simulink model "modelo_q1_fk"  (R2016a)
settings: Solver=VariableStepAuto  StartTime=0.0  StopTime=20  MaxStep=0.001  RelTol=1e-3
values from neighbouring files (symbols this model uses):
  Cm = [1 0 0; 0 1 0]    [gazebo_parameters.m]    (also in gpc.m = [C zeros(ny,1)]; kalman_filter.m)
  Dmsim = zeros(2,1)    [gazebo_parameters.m]    (also in kalman_filter.m = zeros(2,2))
  Kd = dlqr(Amd, Bmd,eye(3),0.7)    [gazebo_parameters.m]    (also in gpc.m = dlqr(A, B, eye(3),1); kalman_filter.m; questao1.m = dlqr(Ad,Bd,Q,R))
  Lkf = dlqr(Amd',Cm',1e-4*eye(3),1*eye(2))'    [gazebo_parameters.m]    (also in kalman_filter.m)
  Pam = 1e8*eye(3)    [gazebo_parameters.m]    (also in kalman_filter.m = 1e-6*eye(3))
  Tsm = 0.005    [gazebo_parameters.m]    (also in kalman_filter.m)
  v = [v1 v2]'    [controledesacoplante.m]    (also in gazebo_parameters.m = 1e-7*eye(2); kalman_filter.m = 1e-8*eye(2); v(1,1) = 1e-0*v(1,1); v(2,2) = 1e-0*v(2,2))
  w = 1e-4*eye(3)    [gazebo_parameters.m]    (also in kalman_filter.m = 1e-10*eye(3); w(1,1) = 1e-0*w(1,1); w(2,2) = 1e-0*w(2,2); w()
  x0m = [0 0 0]    [gazebo_parameters.m]    (also in kalman_filter.m)
undefined symbols (not defined in the file or in its folder): Amd, Bmd, Discrete, sigbuilder_block, Time
libraries: simulink x10, ctrlSharedLib x1
settings Model: Creator=Regner  LastModifiedBy=Regner

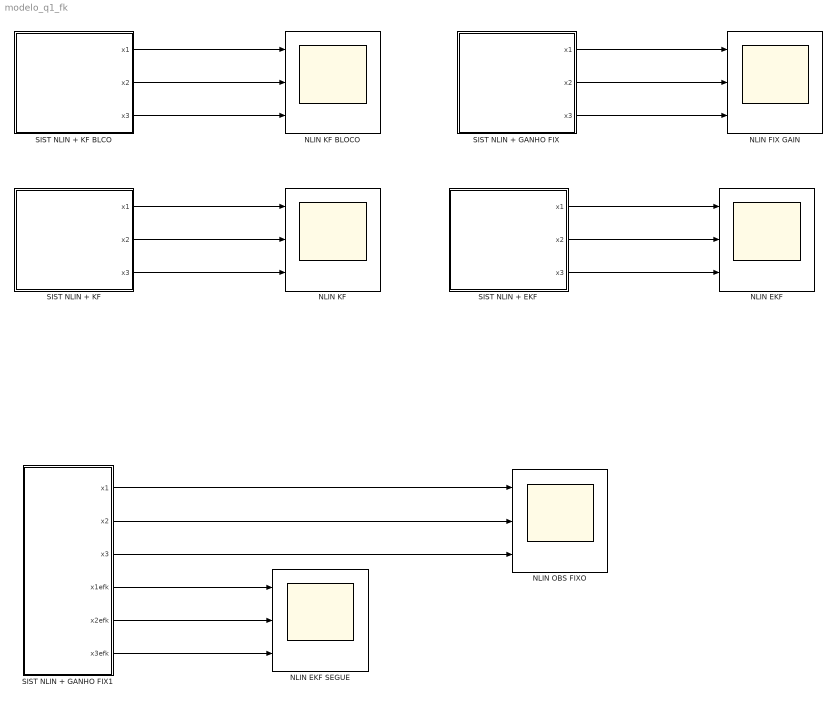
== system modelo_q1_fk ==
  NLIN EKF : Scope  NumInputPorts=3
  NLIN EKF SEGUE : Scope  NumInputPorts=3
  NLIN FIX GAIN : Scope  NumInputPorts=3
  NLIN KF : Scope  NumInputPorts=3
  NLIN KF BLOCO : Scope  NumInputPorts=3
  NLIN OBS FIXO : Scope  NumInputPorts=3
  SIST NLIN + EKF : Subsystem
  SIST NLIN + GANHO FIX : Subsystem
  SIST NLIN + GANHO FIX1 : Subsystem
  SIST NLIN + KF : Subsystem
  SIST NLIN + KF BLCO : Subsystem
  wires:
  SIST NLIN + KF/1(x1) -> NLIN KF/1
  SIST NLIN + KF/2(x2) -> NLIN KF/2
  SIST NLIN + KF/3(x3) -> NLIN KF/3
  SIST NLIN + KF BLCO/1(x1) -> NLIN KF BLOCO/1
  SIST NLIN + KF BLCO/2(x2) -> NLIN KF BLOCO/2
  SIST NLIN + KF BLCO/3(x3) -> NLIN KF BLOCO/3
  SIST NLIN + GANHO FIX/1(x1) -> NLIN FIX GAIN/1
  SIST NLIN + GANHO FIX/2(x2) -> NLIN FIX GAIN/2
  SIST NLIN + GANHO FIX/3(x3) -> NLIN FIX GAIN/3
  SIST NLIN + EKF/2(x2) -> NLIN EKF/2
  SIST NLIN + EKF/3(x3) -> NLIN EKF/3
  SIST NLIN + EKF/1(x1) -> NLIN EKF/1
  SIST NLIN + GANHO FIX1/1(x1) -> NLIN OBS FIXO/1
  SIST NLIN + GANHO FIX1/2(x2) -> NLIN OBS FIXO/2
  SIST NLIN + GANHO FIX1/3(x3) -> NLIN OBS FIXO/3
  SIST NLIN + GANHO FIX1/4(x1efk) -> NLIN EKF SEGUE/1
  SIST NLIN + GANHO FIX1/5(x2efk) -> NLIN EKF SEGUE/2
  SIST NLIN + GANHO FIX1/6(x3efk) -> NLIN EKF SEGUE/3

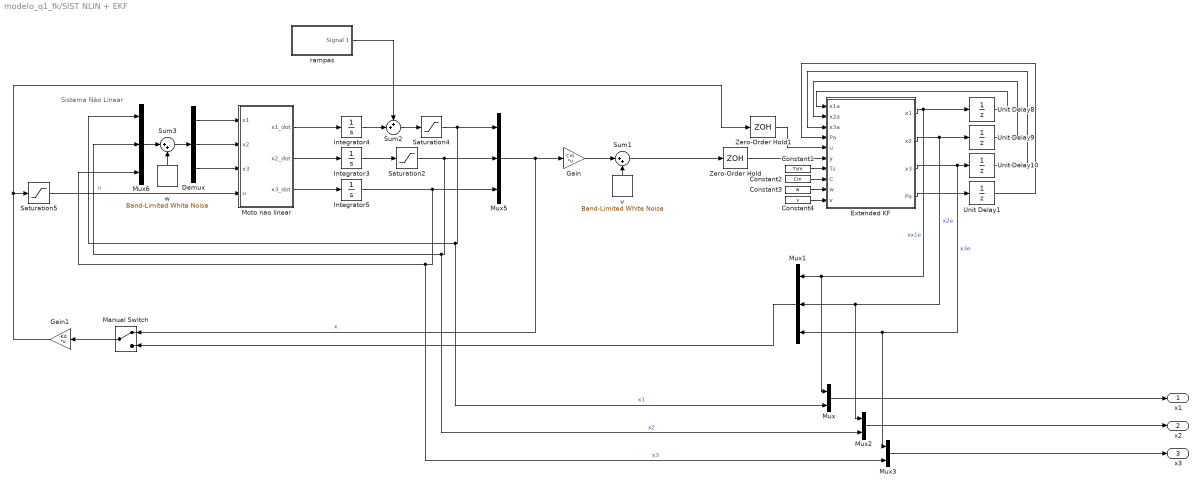
== system modelo_q1_fk/SIST NLIN + EKF ==
  note: Sistema Não Linear
  Constant1 : Constant  Value=Tsm
  Constant2 : Constant  Value=Cm
  Constant3 : Constant  Value=w
  Constant4 : Constant  Value=v
  Demux : Demux  Outputs=3
  Extended KF : MATLAB Function  TreatAsAtomicUnit=on
  Gain : Gain  Gain=Cm  Multiplication=Matrix(K*u)
  Gain1 : Gain  Gain=-Kd  Multiplication=Matrix(K*u)
  Integrator3 : Integrator  InitialCondition=x0m(2)
  Integrator4 : Integrator  InitialCondition=x0m(1)
  Integrator5 : Integrator  InitialCondition=x0m(3)
  Manual Switch : ManualSwitch
  Moto nao linear : MATLAB Function  TreatAsAtomicUnit=on
  Mux : Mux  Inputs=2
  Mux1 : Mux  Inputs=3
  Mux2 : Mux  Inputs=2
  Mux3 : Mux  Inputs=2
  Mux5 : Mux  Inputs=3
  Mux6 : Mux  Inputs=3
  Saturation2 : Saturate  UpperLimit=pi/4  LowerLimit=-pi/4
  Saturation4 : Saturate  UpperLimit=pi/4  LowerLimit=-pi/4
  Saturation5 : Saturate  UpperLimit=pi/2  LowerLimit=-pi/2
  Sum1 : Sum  Inputs=|++
  Sum2 : Sum  Inputs=++|
  Sum3 : Sum  Inputs=|++
  Unit Delay1 : UnitDelay  InitialCondition=Pam  SampleTime=Tsm
  Unit Delay10 : UnitDelay  InitialCondition=x0m(3)  SampleTime=Tsm
  Unit Delay8 : UnitDelay  InitialCondition=x0m(1)  SampleTime=Tsm
  Unit Delay9 : UnitDelay  InitialCondition=x0m(2)  SampleTime=Tsm
  Zero-Order Hold : ZeroOrderHold  SampleTime=Tsm
  Zero-Order Hold1 : ZeroOrderHold  SampleTime=Tsm
  rampas : Subsystem  Tag=STV Subsys  LoadFcn=sigbuilder_block('load');  StartFcn=sigbuilder_block('start');  StopFcn=sigbuilder_block('stop');  ClipboardFcn=sigbuilder_block('clipboard');  mask(Sigbuilder block){}
      mask help: Simulink:masks:SigbuilderBlock_MD
      mask init:
      | if ~strcmp(get_param(bdroot(gcbh),'SimulationStatus'),'stopped') tuvar = sigbuilder_block('maskInit'); end
      settings: CopyFcn=sigbuilder_block('copy');  DeleteFcn=sigbuilder_block('delete');  ModelCloseFcn=sigbuilder_block('modelClose');  PreSaveFcn=sigbuilder_block('preSave');  PauseFcn=sigbuilder_block('pause');  ContinueFcn=sigbuilder_block('continue');  NameChangeFcn=sigbuilder_block('namechange');  OpenFcn=sigbuilder_block('open',[5.4 5.4 1141.2 580.8 ]);  CloseFcn=sigbuilder_block('close');
      mask Display: plot(0, 0, 100, 100,[2, 2, 32, 32, 2], [68, 8, 8, 68, 68],[32, 2], [38, 38], [32, 19, 2],[53, 60, 44], [32, 17, 17, 2],[16, 16, 31, 31]);txt = getActiveGroup(gcbh);text(2, 100, txt,'verticalAlignment', 'top');
  v : simulink/Sources/Band-Limited White Noise  Cov=diag(v)  Ts=Tsm  seed=[23341]
  w : simulink/Sources/Band-Limited White Noise  Cov=diag(w)  Ts=Tsm  seed=[23341]
  x1 : Outport
  x2 : Outport  Port=2
  x3 : Outport  Port=3
  wires:
  Mux2/1 -> x2/1
  Gain/1 -> Sum1/1
  Constant3/1 -> Extended KF/9(w)
  v/1 -> Sum1/2
  Gain1/1 -> Saturation5/1, Zero-Order Hold1/1
  Saturation4/1 -> Mux5/1, Mux6/1, Mux/2  "x1"
  Moto nao linear/2(x2_dot) -> Integrator3/1
  Moto nao linear/1(x1_dot) -> Integrator4/1
  Moto nao linear/3(x3_dot) -> Integrator5/1
  Integrator5/1 -> Mux5/3, Mux6/3, Mux3/2  "x3"
  Sum2/1 -> Saturation4/1
  Mux5/1 -> Gain/1, Manual Switch/1  "x"
  Integrator4/1 -> Sum2/2
  Saturation5/1 -> Moto nao linear/4(u)  "u"
  Saturation2/1 -> Mux5/2, Mux6/2, Mux2/2  "x2"
  Integrator3/1 -> Saturation2/1
  rampas/1(Signal 1) -> Sum2/1
  Constant4/1 -> Extended KF/10(v)
  Mux/1 -> x1/1
  Extended KF/4(Pa) -> Unit Delay1/1
  Mux1/1 -> Manual Switch/2
  Constant2/1 -> Extended KF/8(C)
  Zero-Order Hold/1 -> Extended KF/6(y)
  Sum3/1 -> Demux/1
  Manual Switch/1 -> Gain1/1
  Sum1/1 -> Zero-Order Hold/1
  Demux/3 -> Moto nao linear/3(x3)
  Unit Delay1/1 -> Extended KF/4("Pa ")
  Demux/2 -> Moto nao linear/2(x2)
  w/1 -> Sum3/2
  Mux6/1 -> Sum3/1
  Demux/1 -> Moto nao linear/1(x1)
  Mux3/1 -> x3/1
  Extended KF/2(x2) -> Mux1/2, Mux2/1, Unit Delay9/1  "x2e"
  Extended KF/1(x1) -> Mux1/1, Mux/1, Unit Delay8/1  "xx1e"
  Unit Delay10/1 -> Extended KF/3(x3a)
  Unit Delay8/1 -> Extended KF/1(x1a)
  Extended KF/3(x3) -> Mux1/3, Mux3/1, Unit Delay10/1  "x3e"
  Unit Delay9/1 -> Extended KF/2(x2a)
  Constant1/1 -> Extended KF/7(Ts)
  Zero-Order Hold1/1 -> Extended KF/5(u)

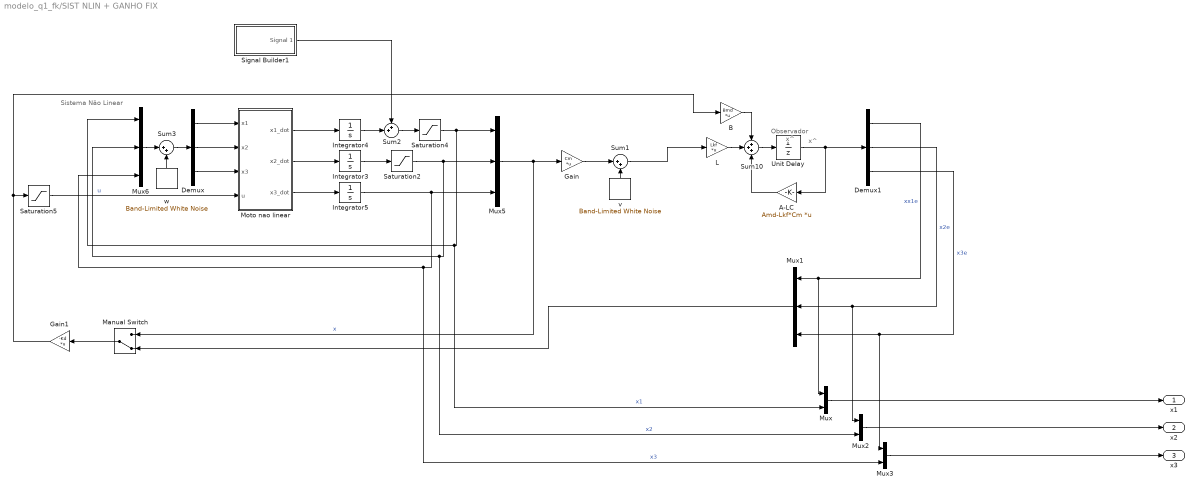
== system modelo_q1_fk/SIST NLIN + GANHO FIX ==
  note: Sistema Não Linear
  note: Observador
  note: x^
  note: x^
  A-LC : Gain  Gain=Amd-Lkf*Cm  Multiplication=Matrix(K*u)
  B : Gain  Gain=Bmd  Multiplication=Matrix(K*u)
  Demux : Demux  Outputs=3
  Demux1 : Demux  Outputs=3
  Gain : Gain  Gain=Cm  Multiplication=Matrix(K*u)
  Gain1 : Gain  Gain=-Kd  Multiplication=Matrix(K*u)
  Integrator3 : Integrator  InitialCondition=x0m(2)
  Integrator4 : Integrator  InitialCondition=x0m(1)
  Integrator5 : Integrator  InitialCondition=x0m(3)
  L : Gain  Gain=Lkf  Multiplication=Matrix(K*u)
  Manual Switch : ManualSwitch  CurrentSetting=0
  Moto nao linear : MATLAB Function  TreatAsAtomicUnit=on
  Mux : Mux  Inputs=2
  Mux1 : Mux  Inputs=3
  Mux2 : Mux  Inputs=2
  Mux3 : Mux  Inputs=2
  Mux5 : Mux  Inputs=3
  Mux6 : Mux  Inputs=3
  Saturation2 : Saturate  UpperLimit=pi/4  LowerLimit=-pi/4
  Saturation4 : Saturate  UpperLimit=pi/4  LowerLimit=-pi/4
  Saturation5 : Saturate  UpperLimit=pi/2  LowerLimit=-pi/2
  Signal Builder1 : Subsystem  Tag=STV Subsys  LoadFcn=sigbuilder_block('load');  StartFcn=sigbuilder_block('start');  StopFcn=sigbuilder_block('stop');  ClipboardFcn=sigbuilder_block('clipboard');  mask(Sigbuilder block){}
      mask help: Simulink:masks:SigbuilderBlock_MD
      mask init:
      | if ~strcmp(get_param(bdroot(gcbh),'SimulationStatus'),'stopped') tuvar = sigbuilder_block('maskInit'); end
      settings: CopyFcn=sigbuilder_block('copy');  DeleteFcn=sigbuilder_block('delete');  ModelCloseFcn=sigbuilder_block('modelClose');  PreSaveFcn=sigbuilder_block('preSave');  PauseFcn=sigbuilder_block('pause');  ContinueFcn=sigbuilder_block('continue');  NameChangeFcn=sigbuilder_block('namechange');  OpenFcn=sigbuilder_block('open',[5.4 5.4 1141.2 580.8 ]);  CloseFcn=sigbuilder_block('close');
      mask Display: plot(0, 0, 100, 100,[2, 2, 32, 32, 2], [68, 8, 8, 68, 68],[32, 2], [38, 38], [32, 19, 2],[53, 60, 44], [32, 17, 17, 2],[16, 16, 31, 31]);txt = getActiveGroup(gcbh);text(2, 100, txt,'verticalAlignment', 'top');
  Sum1 : Sum  Inputs=|++
  Sum10 : Sum  Inputs=+++
  Sum2 : Sum  Inputs=++|
  Sum3 : Sum  Inputs=|++
  Unit Delay : UnitDelay  InitialCondition=x0m  SampleTime=Tsm
  v : simulink/Sources/Band-Limited White Noise  Cov=diag(v)  Ts=Tsm  seed=[23341]
  w : simulink/Sources/Band-Limited White Noise  Cov=diag(w)  Ts=Tsm  seed=[23341]
  x1 : Outport
  x2 : Outport  Port=2
  x3 : Outport  Port=3
  wires:
  Unit Delay/1 -> Demux1/1, A-LC/1
  Gain1/1 -> B/1, Saturation5/1
  Demux1/3 -> Mux3/1, Mux1/3  "x3e"
  Demux1/1 -> Mux/1, Mux1/1  "xx1e"
  Demux1/2 -> Mux2/1, Mux1/2  "x2e"
  Mux3/1 -> x3/1
  Demux/1 -> Moto nao linear/1(x1)
  Mux6/1 -> Sum3/1
  w/1 -> Sum3/2
  Demux/2 -> Moto nao linear/2(x2)
  Demux/3 -> Moto nao linear/3(x3)
  Manual Switch/1 -> Gain1/1
  Sum3/1 -> Demux/1
  Sum1/1 -> L/1
  Mux1/1 -> Manual Switch/2
  Mux/1 -> x1/1
  Signal Builder1/1(Signal 1) -> Sum2/1
  Integrator3/1 -> Saturation2/1
  Saturation2/1 -> Mux2/2, Mux6/2, Mux5/2  "x2"
  Saturation5/1 -> Moto nao linear/4(u)  "u"
  Integrator4/1 -> Sum2/2
  Mux5/1 -> Manual Switch/1, Gain/1  "x"
  Sum2/1 -> Saturation4/1
  Integrator5/1 -> Mux3/2, Mux6/3, Mux5/3  "x3"
  Moto nao linear/3(x3_dot) -> Integrator5/1
  Moto nao linear/1(x1_dot) -> Integrator4/1
  Moto nao linear/2(x2_dot) -> Integrator3/1
  Saturation4/1 -> Mux/2, Mux6/1, Mux5/1  "x1"
  v/1 -> Sum1/2
  Gain/1 -> Sum1/1
  Mux2/1 -> x2/1
  Sum10/1 -> Unit Delay/1
  L/1 -> Sum10/2
  A-LC/1 -> Sum10/3
  B/1 -> Sum10/1

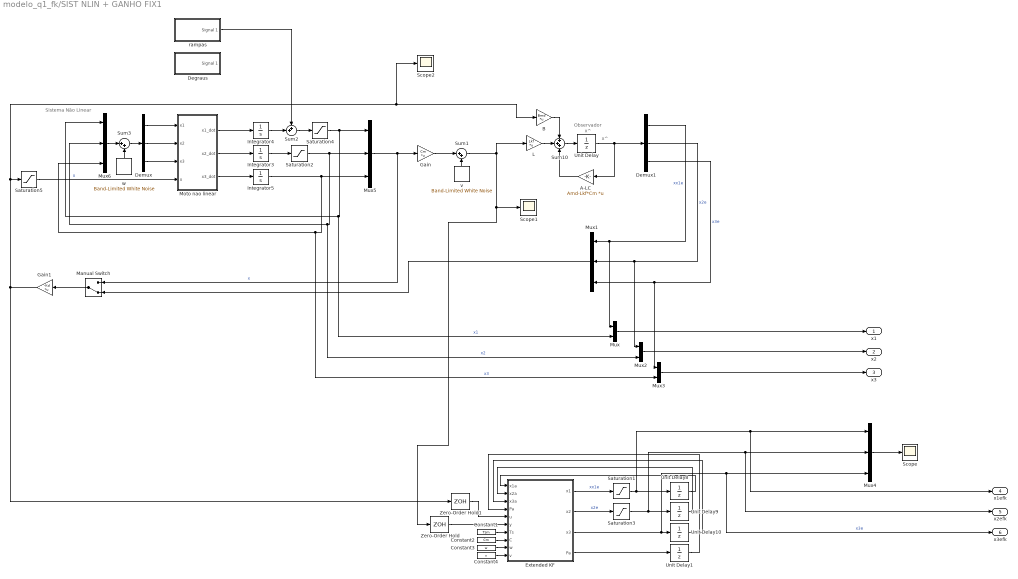
== system modelo_q1_fk/SIST NLIN + GANHO FIX1 ==
  note: x^
  note: x^
  note: Observador
  note: Sistema Não Linear
  A-LC : Gain  Gain=Amd-Lkf*Cm  Multiplication=Matrix(K*u)
  B : Gain  Gain=Bmd  Multiplication=Matrix(K*u)
  Constant1 : Constant  Value=Tsm
  Constant2 : Constant  Value=Cm
  Constant3 : Constant  Value=w
  Constant4 : Constant  Value=v
  Degraus : Subsystem  Tag=STV Subsys  LoadFcn=sigbuilder_block('load');  StartFcn=sigbuilder_block('start');  StopFcn=sigbuilder_block('stop');  ClipboardFcn=sigbuilder_block('clipboard');  mask(Sigbuilder block){}
      mask help: Simulink:masks:SigbuilderBlock_MD
      mask init:
      | if ~strcmp(get_param(bdroot(gcbh),'SimulationStatus'),'stopped') tuvar = sigbuilder_block('maskInit'); end
      settings: CopyFcn=sigbuilder_block('copy');  DeleteFcn=sigbuilder_block('delete');  ModelCloseFcn=sigbuilder_block('modelClose');  PreSaveFcn=sigbuilder_block('preSave');  PauseFcn=sigbuilder_block('pause');  ContinueFcn=sigbuilder_block('continue');  NameChangeFcn=sigbuilder_block('namechange');  OpenFcn=sigbuilder_block('open',[5.4 5.4 1141.2 580.8 ]);  CloseFcn=sigbuilder_block('close');
      mask Display: plot(0, 0, 100, 100,[2, 2, 32, 32, 2], [68, 8, 8, 68, 68],[32, 2], [38, 38], [32, 19, 2],[53, 60, 44], [32, 17, 17, 2],[16, 16, 31, 31]);txt = getActiveGroup(gcbh);text(2, 100, txt,'verticalAlignment', 'top');
  Demux : Demux  Outputs=3
  Demux1 : Demux  Outputs=3
  Extended KF : MATLAB Function  TreatAsAtomicUnit=on
  Gain : Gain  Gain=Cm  Multiplication=Matrix(K*u)
  Gain1 : Gain  Gain=-Kd  Multiplication=Matrix(K*u)
  Integrator3 : Integrator  InitialCondition=x0m(2)
  Integrator4 : Integrator  InitialCondition=x0m(1)
  Integrator5 : Integrator  InitialCondition=x0m(3)
  L : Gain  Gain=Lkf  Multiplication=Matrix(K*u)
  Manual Switch : ManualSwitch  CurrentSetting=0
  Moto nao linear : MATLAB Function  TreatAsAtomicUnit=on
  Mux : Mux  Inputs=2
  Mux{1,4..6} (4 alike) : Mux  Inputs=3
  Mux2 : Mux  Inputs=2
  Mux3 : Mux  Inputs=2
  Saturation{1..4} (4 alike) : Saturate  UpperLimit=pi/4  LowerLimit=-pi/4
  Saturation5 : Saturate  UpperLimit=pi/2  LowerLimit=-pi/2
  Scope : Scope
  Scope1 : Scope
  Scope2 : Scope
  Sum1 : Sum  Inputs=|++
  Sum10 : Sum  Inputs=+++
  Sum2 : Sum  Inputs=++|
  Sum3 : Sum  Inputs=|++
  Unit Delay : UnitDelay  InitialCondition=x0m  SampleTime=Tsm
  Unit Delay1 : UnitDelay  InitialCondition=Pam  SampleTime=Tsm
  Unit Delay10 : UnitDelay  InitialCondition=x0m(3)  SampleTime=Tsm
  Unit Delay8 : UnitDelay  InitialCondition=x0m(1)  SampleTime=Tsm
  Unit Delay9 : UnitDelay  InitialCondition=x0m(2)  SampleTime=Tsm
  Zero-Order Hold : ZeroOrderHold  SampleTime=Tsm
  Zero-Order Hold1 : ZeroOrderHold  SampleTime=Tsm
  rampas : Subsystem  Tag=STV Subsys  LoadFcn=sigbuilder_block('load');  StartFcn=sigbuilder_block('start');  StopFcn=sigbuilder_block('stop');  ClipboardFcn=sigbuilder_block('clipboard');  mask(Sigbuilder block){}
      mask help: Simulink:masks:SigbuilderBlock_MD
      mask init:
      | if ~strcmp(get_param(bdroot(gcbh),'SimulationStatus'),'stopped') tuvar = sigbuilder_block('maskInit'); end
      settings: CopyFcn=sigbuilder_block('copy');  DeleteFcn=sigbuilder_block('delete');  ModelCloseFcn=sigbuilder_block('modelClose');  PreSaveFcn=sigbuilder_block('preSave');  PauseFcn=sigbuilder_block('pause');  ContinueFcn=sigbuilder_block('continue');  NameChangeFcn=sigbuilder_block('namechange');  OpenFcn=sigbuilder_block('open',[5.4 5.4 1141.2 580.8 ]);  CloseFcn=sigbuilder_block('close');
      mask Display: plot(0, 0, 100, 100,[2, 2, 32, 32, 2], [68, 8, 8, 68, 68],[32, 2], [38, 38], [32, 19, 2],[53, 60, 44], [32, 17, 17, 2],[16, 16, 31, 31]);txt = getActiveGroup(gcbh);text(2, 100, txt,'verticalAlignment', 'top');
  v : simulink/Sources/Band-Limited White Noise  Cov=diag(v)  Ts=Tsm  seed=[23341]
  w : simulink/Sources/Band-Limited White Noise  Cov=diag(w)  Ts=Tsm  seed=[23341]
  x1 : Outport
  x2 : Outport  Port=2
  x3 : Outport  Port=3
  x1efk : Outport  Port=4
  x2efk : Outport  Port=5
  x3efk : Outport  Port=6
  wires:
  B/1 -> Sum10/1
  A-LC/1 -> Sum10/3
  L/1 -> Sum10/2
  Sum10/1 -> Unit Delay/1
  Mux2/1 -> x2/1
  Gain/1 -> Sum1/1
  v/1 -> Sum1/2
  Saturation4/1 -> Mux5/1, Mux6/1, Mux/2  "x1"
  Moto nao linear/2(x2_dot) -> Integrator3/1
  Moto nao linear/1(x1_dot) -> Integrator4/1
  Moto nao linear/3(x3_dot) -> Integrator5/1
  Integrator5/1 -> Mux5/3, Mux6/3, Mux3/2  "x3"
  Sum2/1 -> Saturation4/1
  Mux5/1 -> Gain/1, Manual Switch/1  "x"
  Integrator4/1 -> Sum2/2
  Saturation5/1 -> Moto nao linear/4(u)  "u"
  Saturation2/1 -> Mux5/2, Mux6/2, Mux2/2  "x2"
  Integrator3/1 -> Saturation2/1
  rampas/1(Signal 1) -> Sum2/1
  Mux/1 -> x1/1
  Mux1/1 -> Manual Switch/2
  Sum1/1 -> L/1, Scope1/1, Zero-Order Hold/1
  Sum3/1 -> Demux/1
  Manual Switch/1 -> Gain1/1
  Demux/3 -> Moto nao linear/3(x3)
  Demux/2 -> Moto nao linear/2(x2)
  w/1 -> Sum3/2
  Mux6/1 -> Sum3/1
  Demux/1 -> Moto nao linear/1(x1)
  Mux3/1 -> x3/1
  Demux1/2 -> Mux1/2, Mux2/1  "x2e"
  Demux1/1 -> Mux1/1, Mux/1  "xx1e"
  Demux1/3 -> Mux1/3, Mux3/1  "x3e"
  Gain1/1 -> Saturation5/1, Scope2/1, B/1, Zero-Order Hold1/1
  Unit Delay/1 -> A-LC/1, Demux1/1
  Constant3/1 -> Extended KF/9(w)
  Constant4/1 -> Extended KF/10(v)
  Extended KF/4(Pa) -> Unit Delay1/1
  Constant2/1 -> Extended KF/8(C)
  Zero-Order Hold/1 -> Extended KF/6(y)
  Unit Delay1/1 -> Extended KF/4("Pa ")
  Extended KF/2(x2) -> Saturation3/1  "x2e"
  Extended KF/1(x1) -> Saturation1/1  "xx1e"
  Unit Delay10/1 -> Extended KF/3(x3a)
  Unit Delay8/1 -> Extended KF/1(x1a)
  Extended KF/3(x3) -> x3efk/1, Mux4/3, Unit Delay10/1  "x3e"
  Unit Delay9/1 -> Extended KF/2(x2a)
  Constant1/1 -> Extended KF/7(Ts)
  Zero-Order Hold1/1 -> Extended KF/5(u)
  Mux4/1 -> Scope/1
  Saturation1/1 -> x1efk/1, Mux4/1, Unit Delay8/1
  Saturation3/1 -> x2efk/1, Mux4/2, Unit Delay9/1

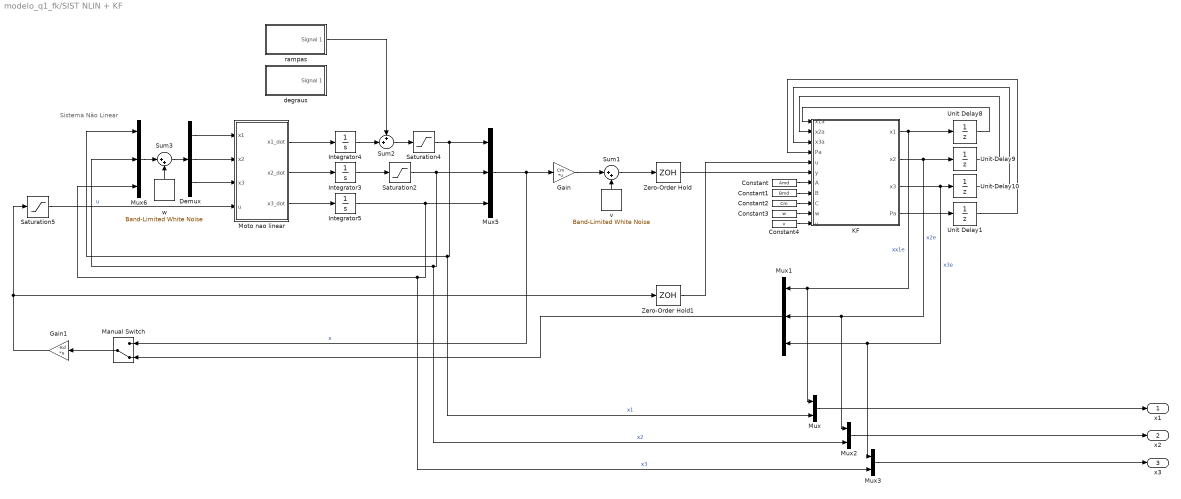
== system modelo_q1_fk/SIST NLIN + KF ==
  note: Sistema Não Linear
  Constant : Constant  Value=Amd
  Constant1 : Constant  Value=Bmd
  Constant2 : Constant  Value=Cm
  Constant3 : Constant  Value=w
  Constant4 : Constant  Value=v
  Demux : Demux  Outputs=3
  Gain : Gain  Gain=Cm  Multiplication=Matrix(K*u)
  Gain1 : Gain  Gain=-Kd  Multiplication=Matrix(K*u)
  Integrator3 : Integrator  InitialCondition=x0m(2)
  Integrator4 : Integrator  InitialCondition=x0m(1)
  Integrator5 : Integrator  InitialCondition=x0m(3)
  KF : MATLAB Function  TreatAsAtomicUnit=on
  Manual Switch : ManualSwitch  CurrentSetting=0
  Moto nao linear : MATLAB Function  TreatAsAtomicUnit=on
  Mux : Mux  Inputs=2
  Mux1 : Mux  Inputs=3
  Mux2 : Mux  Inputs=2
  Mux3 : Mux  Inputs=2
  Mux5 : Mux  Inputs=3
  Mux6 : Mux  Inputs=3
  Saturation2 : Saturate  UpperLimit=pi/4  LowerLimit=-pi/4
  Saturation4 : Saturate  UpperLimit=pi/4  LowerLimit=-pi/4
  Saturation5 : Saturate  UpperLimit=pi/2  LowerLimit=-pi/2
  Sum1 : Sum  Inputs=|++
  Sum2 : Sum  Inputs=++|
  Sum3 : Sum  Inputs=|++
  Unit Delay1 : UnitDelay  InitialCondition=Pam  SampleTime=Tsm
  Unit Delay10 : UnitDelay  InitialCondition=x0m(3)  SampleTime=Tsm
  Unit Delay8 : UnitDelay  InitialCondition=x0m(1)  SampleTime=Tsm
  Unit Delay9 : UnitDelay  InitialCondition=x0m(2)  SampleTime=Tsm
  Zero-Order Hold : ZeroOrderHold  SampleTime=Tsm
  Zero-Order Hold1 : ZeroOrderHold  SampleTime=Tsm
  degraus : Subsystem  Tag=STV Subsys  LoadFcn=sigbuilder_block('load');  StartFcn=sigbuilder_block('start');  StopFcn=sigbuilder_block('stop');  ClipboardFcn=sigbuilder_block('clipboard');  mask(Sigbuilder block){}
      mask help: Simulink:masks:SigbuilderBlock_MD
      mask init:
      | if ~strcmp(get_param(bdroot(gcbh),'SimulationStatus'),'stopped') tuvar = sigbuilder_block('maskInit'); end
      settings: CopyFcn=sigbuilder_block('copy');  DeleteFcn=sigbuilder_block('delete');  ModelCloseFcn=sigbuilder_block('modelClose');  PreSaveFcn=sigbuilder_block('preSave');  PauseFcn=sigbuilder_block('pause');  ContinueFcn=sigbuilder_block('continue');  NameChangeFcn=sigbuilder_block('namechange');  OpenFcn=sigbuilder_block('open',[5.4 5.4 1141.2 580.8 ]);  CloseFcn=sigbuilder_block('close');
      mask Display: plot(0, 0, 100, 100,[2, 2, 32, 32, 2], [68, 8, 8, 68, 68],[32, 2], [38, 38], [32, 19, 2],[53, 60, 44], [32, 17, 17, 2],[16, 16, 31, 31]);txt = getActiveGroup(gcbh);text(2, 100, txt,'verticalAlignment', 'top');
  rampas : Subsystem  Tag=STV Subsys  LoadFcn=sigbuilder_block('load');  StartFcn=sigbuilder_block('start');  StopFcn=sigbuilder_block('stop');  ClipboardFcn=sigbuilder_block('clipboard');  mask(Sigbuilder block){}
      mask help: Simulink:masks:SigbuilderBlock_MD
      mask init:
      | if ~strcmp(get_param(bdroot(gcbh),'SimulationStatus'),'stopped') tuvar = sigbuilder_block('maskInit'); end
      settings: CopyFcn=sigbuilder_block('copy');  DeleteFcn=sigbuilder_block('delete');  ModelCloseFcn=sigbuilder_block('modelClose');  PreSaveFcn=sigbuilder_block('preSave');  PauseFcn=sigbuilder_block('pause');  ContinueFcn=sigbuilder_block('continue');  NameChangeFcn=sigbuilder_block('namechange');  OpenFcn=sigbuilder_block('open',[5.4 5.4 1141.2 580.8 ]);  CloseFcn=sigbuilder_block('close');
      mask Display: plot(0, 0, 100, 100,[2, 2, 32, 32, 2], [68, 8, 8, 68, 68],[32, 2], [38, 38], [32, 19, 2],[53, 60, 44], [32, 17, 17, 2],[16, 16, 31, 31]);txt = getActiveGroup(gcbh);text(2, 100, txt,'verticalAlignment', 'top');
  v : simulink/Sources/Band-Limited White Noise  Cov=diag(v)  Ts=Tsm  seed=[23341]
  w : simulink/Sources/Band-Limited White Noise  Cov=diag(w)  Ts=Tsm  seed=[23341]
  x1 : Outport
  x2 : Outport  Port=2
  x3 : Outport  Port=3
  wires:
  Unit Delay9/1 -> KF/2(x2a)
  KF/3(x3) -> Mux3/1, Mux1/3, Unit Delay10/1  "x3e"
  Unit Delay8/1 -> KF/1(x1a)
  Unit Delay10/1 -> KF/3(x3a)
  KF/1(x1) -> Mux/1, Mux1/1, Unit Delay8/1  "xx1e"
  KF/2(x2) -> Mux2/1, Mux1/2, Unit Delay9/1  "x2e"
  Mux3/1 -> x3/1
  Demux/1 -> Moto nao linear/1(x1)
  Mux6/1 -> Sum3/1
  w/1 -> Sum3/2
  Demux/2 -> Moto nao linear/2(x2)
  Unit Delay1/1 -> KF/4("Pa ")
  Demux/3 -> Moto nao linear/3(x3)
  Sum1/1 -> Zero-Order Hold/1
  Manual Switch/1 -> Gain1/1
  Sum3/1 -> Demux/1
  Zero-Order Hold/1 -> KF/6(y)
  Constant2/1 -> KF/9(C)
  Mux1/1 -> Manual Switch/2
  KF/4(Pa) -> Unit Delay1/1
  Mux/1 -> x1/1
  Constant/1 -> KF/7(A)
  Constant4/1 -> KF/11(v)
  rampas/1(Signal 1) -> Sum2/1
  Integrator3/1 -> Saturation2/1
  Saturation2/1 -> Mux2/2, Mux6/2, Mux5/2  "x2"
  Saturation5/1 -> Moto nao linear/4(u)  "u"
  Integrator4/1 -> Sum2/2
  Mux5/1 -> Manual Switch/1, Gain/1  "x"
  Sum2/1 -> Saturation4/1
  Integrator5/1 -> Mux3/2, Mux6/3, Mux5/3  "x3"
  Moto nao linear/3(x3_dot) -> Integrator5/1
  Moto nao linear/1(x1_dot) -> Integrator4/1
  Moto nao linear/2(x2_dot) -> Integrator3/1
  Saturation4/1 -> Mux/2, Mux6/1, Mux5/1  "x1"
  Gain1/1 -> Saturation5/1, Zero-Order Hold1/1
  v/1 -> Sum1/2
  Constant1/1 -> KF/8(B)
  Constant3/1 -> KF/10(w)
  Gain/1 -> Sum1/1
  Mux2/1 -> x2/1
  Zero-Order Hold1/1 -> KF/5(u)

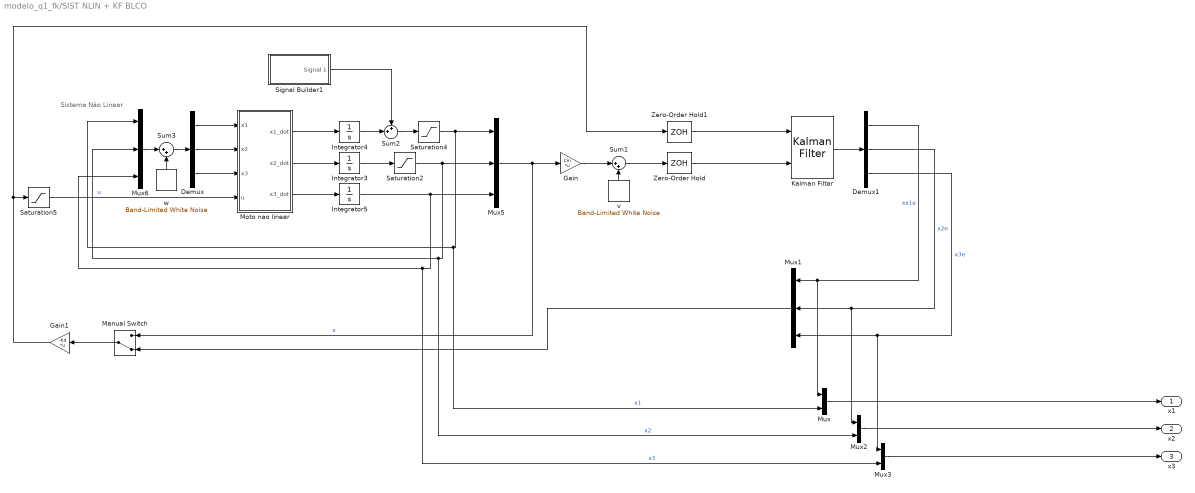
== system modelo_q1_fk/SIST NLIN + KF BLCO ==
  note: Sistema Não Linear
  Demux : Demux  Outputs=3
  Demux1 : Demux  Outputs=3
  Gain : Gain  Gain=Cm  Multiplication=Matrix(K*u)
  Gain1 : Gain  Gain=-Kd  Multiplication=Matrix(K*u)
  Integrator3 : Integrator  InitialCondition=x0m(2)
  Integrator4 : Integrator  InitialCondition=x0m(1)
  Integrator5 : Integrator  InitialCondition=x0m(3)
  Kalman Filter : ctrlSharedLib/Kalman Filter  TimeDomain=Discrete-Time  UseCurrentEstimator=on  ModelSource=Individual A, B, C, D matrices  ModelSourceVariable=ss(Amd,Bmd,Cm,Dmsim)  A=Amd  B=Bmd  C=Cm  D=zeros(2,1)  NumberOfStates=3  NumberOfInputs=1  NumberOfOutputs=2  InitialEstimateSource=Dialog  X0=x0m  P0=10  UseK=off  UseGH=off  NumberOfProcessNoiseInputs=1  G=1  TimeInvariantG=on  H=0  TimeInvariantH=on  Q=w*1e4  TimeInvariantQ=on  R=v*1e4  TimeInvariantR=on  N=0  TimeInvariantN=on  AddInputPort=on  AddEnablePort=off  OutputEstimatedY=off  OutputP=off  Ts=Tsm
  Manual Switch : ManualSwitch  CurrentSetting=0
  Moto nao linear : MATLAB Function  TreatAsAtomicUnit=on
  Mux : Mux  Inputs=2
  Mux1 : Mux  Inputs=3
  Mux2 : Mux  Inputs=2
  Mux3 : Mux  Inputs=2
  Mux5 : Mux  Inputs=3
  Mux6 : Mux  Inputs=3
  Saturation2 : Saturate  UpperLimit=pi/4  LowerLimit=-pi/4
  Saturation4 : Saturate  UpperLimit=pi/4  LowerLimit=-pi/4
  Saturation5 : Saturate  UpperLimit=pi/2  LowerLimit=-pi/2
  Signal Builder1 : Subsystem  Tag=STV Subsys  LoadFcn=sigbuilder_block('load');  StartFcn=sigbuilder_block('start');  StopFcn=sigbuilder_block('stop');  ClipboardFcn=sigbuilder_block('clipboard');  mask(Sigbuilder block){}
      mask help: Simulink:masks:SigbuilderBlock_MD
      mask init:
      | if ~strcmp(get_param(bdroot(gcbh),'SimulationStatus'),'stopped') tuvar = sigbuilder_block('maskInit'); end
      settings: CopyFcn=sigbuilder_block('copy');  DeleteFcn=sigbuilder_block('delete');  ModelCloseFcn=sigbuilder_block('modelClose');  PreSaveFcn=sigbuilder_block('preSave');  PauseFcn=sigbuilder_block('pause');  ContinueFcn=sigbuilder_block('continue');  NameChangeFcn=sigbuilder_block('namechange');  OpenFcn=sigbuilder_block('open',[5.4 5.4 1141.2 580.8 ]);  CloseFcn=sigbuilder_block('close');
      mask Display: plot(0, 0, 100, 100,[2, 2, 32, 32, 2], [68, 8, 8, 68, 68],[32, 2], [38, 38], [32, 19, 2],[53, 60, 44], [32, 17, 17, 2],[16, 16, 31, 31]);txt = getActiveGroup(gcbh);text(2, 100, txt,'verticalAlignment', 'top');
  Sum1 : Sum  Inputs=|++
  Sum2 : Sum  Inputs=++|
  Sum3 : Sum  Inputs=|++
  Zero-Order Hold : ZeroOrderHold  SampleTime=Tsm
  Zero-Order Hold1 : ZeroOrderHold  SampleTime=Tsm
  v : simulink/Sources/Band-Limited White Noise  Cov=diag(v)  Ts=Tsm  seed=[23341]
  w : simulink/Sources/Band-Limited White Noise  Cov=diag(w)  Ts=Tsm  seed=[23341]
  x1 : Outport
  x2 : Outport  Port=2
  x3 : Outport  Port=3
  wires:
  Mux2/1 -> x2/1
  Gain/1 -> Sum1/1
  v/1 -> Sum1/2
  Gain1/1 -> Zero-Order Hold1/1, Saturation5/1
  Saturation4/1 -> Mux5/1, Mux6/1, Mux/2  "x1"
  Moto nao linear/2(x2_dot) -> Integrator3/1
  Moto nao linear/1(x1_dot) -> Integrator4/1
  Moto nao linear/3(x3_dot) -> Integrator5/1
  Integrator5/1 -> Mux5/3, Mux6/3, Mux3/2  "x3"
  Sum2/1 -> Saturation4/1
  Mux5/1 -> Gain/1, Manual Switch/1  "x"
  Integrator4/1 -> Sum2/2
  Saturation5/1 -> Moto nao linear/4(u)  "u"
  Saturation2/1 -> Mux5/2, Mux6/2, Mux2/2  "x2"
  Integrator3/1 -> Saturation2/1
  Signal Builder1/1(Signal 1) -> Sum2/1
  Mux/1 -> x1/1
  Mux1/1 -> Manual Switch/2
  Zero-Order Hold/1 -> Kalman Filter/2
  Sum3/1 -> Demux/1
  Manual Switch/1 -> Gain1/1
  Sum1/1 -> Zero-Order Hold/1
  Demux/3 -> Moto nao linear/3(x3)
  Demux/2 -> Moto nao linear/2(x2)
  w/1 -> Sum3/2
  Mux6/1 -> Sum3/1
  Demux/1 -> Moto nao linear/1(x1)
  Mux3/1 -> x3/1
  Demux1/2 -> Mux1/2, Mux2/1  "x2e"
  Demux1/1 -> Mux1/1, Mux/1  "xx1e"
  Demux1/3 -> Mux1/3, Mux3/1  "x3e"
  Zero-Order Hold1/1 -> Kalman Filter/1
  Kalman Filter/1 -> Demux1/1

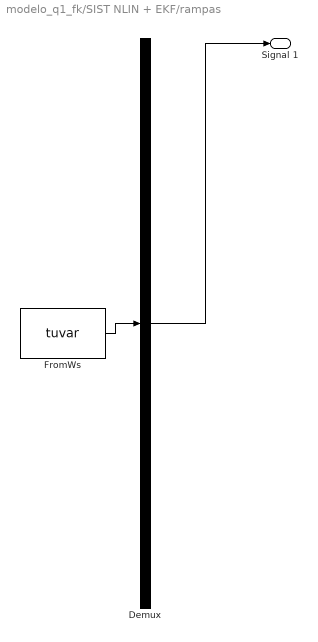
== system modelo_q1_fk/SIST NLIN + EKF/rampas ==
  Demux : Demux  Tag=STV Demux  Outputs=1
  FromWs : FromWorkspace  Tag=STV FromWs  VariableName=tuvar  SampleTime=0
      SigBuilderData=|
      | common.afterFinalStr = 'Extrapolate'
      | common.sampleTime = 0
      | dataSet.timeRange = [0 20]
      | dataSet.name = 'Group 1'
      | sbobj.Groups.Name = 'Group 1'
      | sbobj.Groups.Signals.Name = 'Signal 1'
      | sbobj.Groups.Signals.XData = [0 1.8 2 3.1 3.3 3.9 5 5.8 5.8 6.1 6.1 6.75 10.45 10.45 11.6 11.6 12.6 12.6 13.5 13.5 14.6 14.75 17.95 17.95 18.15 18.6 20]
      | sbobj.Groups.Signals.YData = [-0.01 -0.01 0 0.325 0.615 -0.05 0.2 0.51 0.53 0.53 0.515 -0.14 -0.045 -0.04 0.005 0 -0.045 -0.04 -0.015 -0.02 -0.42 -0.42 0.595 0.61 0.61 0.03 0.03]
      | sbobj.Groups.TimeRange = [0 20]
  Signal 1 : Outport  Tag=STV Outport
  wires:
  FromWs/1 -> Demux/1
  Demux/1 -> Signal 1/1

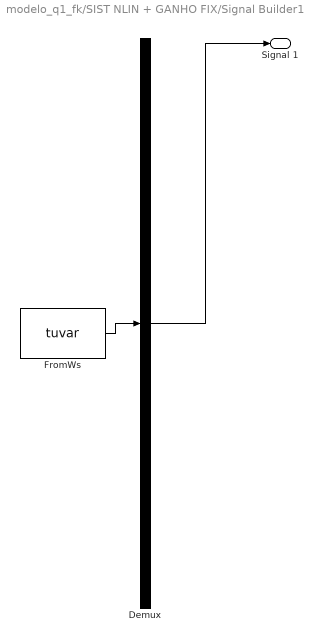
== system modelo_q1_fk/SIST NLIN + GANHO FIX/Signal Builder1 ==
  Demux : Demux  Tag=STV Demux  Outputs=1
  FromWs : FromWorkspace  Tag=STV FromWs  VariableName=tuvar  SampleTime=0
      SigBuilderData=|
      | common.afterFinalStr = 'Extrapolate'
      | common.sampleTime = 0
      | dataSet.timeRange = [0 20]
      | dataSet.name = 'Group 1'
      | sbobj.Groups.Name = 'Group 1'
      | sbobj.Groups.Signals.Name = 'Signal 1'
      | sbobj.Groups.Signals.XData = [0 1.8 3.1 3.1 3.3 3.3 3.9 3.9 5.8 5.8 6.1 6.1 6.75 6.75 10.45 10.45 11.6 11.6 12.6 12.6 13.5 13.5 14.6 14.6 14.75 14.75 17.95 17.95 18.15 18.15 18.6 20]
      | sbobj.Groups.Signals.YData = [-0.01 -0.01 -0.01 0.695 0.695 -0.05 -0.05 0 0 0.53 0.53 -0.01 -0.01 -0.14 -0.14 -0.04 -0.04 0 0 -0.04 -0.04 -0.02 -0.02 -0.42 -0.42 -0.01 -0.01 0.61 0.61 0.03 0.03 0.03]
      | sbobj.Groups.TimeRange = [0 20]
  Signal 1 : Outport  Tag=STV Outport
  wires:
  Demux/1 -> Signal 1/1
  FromWs/1 -> Demux/1

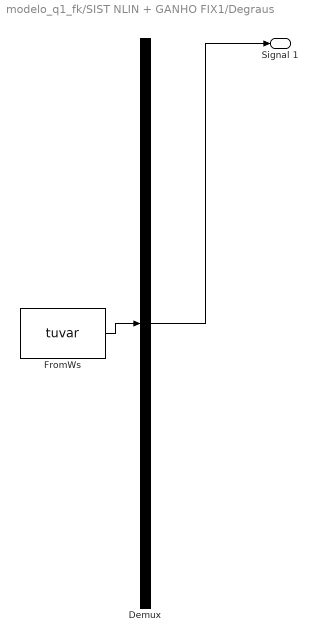
== system modelo_q1_fk/SIST NLIN + GANHO FIX1/Degraus ==
  Demux : Demux  Tag=STV Demux  Outputs=1
  FromWs : FromWorkspace  Tag=STV FromWs  VariableName=tuvar  SampleTime=0
      SigBuilderData=|
      | common.afterFinalStr = 'Extrapolate'
      | common.sampleTime = 0
      | dataSet.timeRange = [0 20]
      | dataSet.name = 'Group 1'
      | sbobj.Groups.Name = 'Group 1'
      | sbobj.Groups.Signals.Name = 'Signal 1'
      | sbobj.Groups.Signals.XData = [0 1.8 3.1 3.1 3.3 3.3 3.9 3.9 5.8 5.8 6.1 6.1 6.75 6.75 10.45 10.45 11.6 11.6 12.6 12.6 13.5 13.5 14.6 14.6 14.75 14.75 17.95 17.95 18.15 18.15 18.6 20]
      | sbobj.Groups.Signals.YData = [-0.01 -0.01 -0.01 0.695 0.695 -0.05 -0.05 0 0 0.53 0.53 -0.01 -0.01 -0.14 -0.14 -0.04 -0.04 0 0 -0.04 -0.04 -0.02 -0.02 -0.42 -0.42 -0.01 -0.01 0.61 0.61 0.03 0.03 0.03]
      | sbobj.Groups.TimeRange = [0 20]
  Signal 1 : Outport  Tag=STV Outport
  wires:
  FromWs/1 -> Demux/1
  Demux/1 -> Signal 1/1

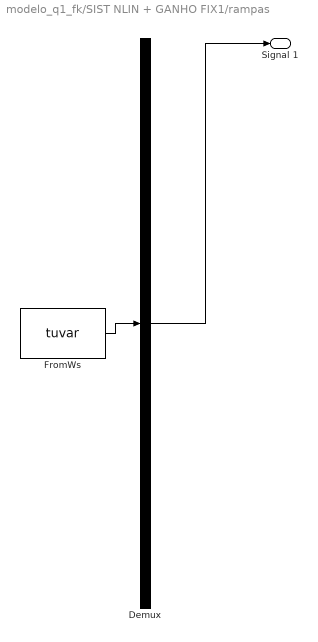
== system modelo_q1_fk/SIST NLIN + GANHO FIX1/rampas ==
  Demux : Demux  Tag=STV Demux  Outputs=1
  FromWs : FromWorkspace  Tag=STV FromWs  VariableName=tuvar  SampleTime=0
      SigBuilderData=|
      | common.afterFinalStr = 'Extrapolate'
      | common.sampleTime = 0
      | dataSet.timeRange = [0 20]
      | dataSet.name = 'Group 1'
      | sbobj.Groups.Name = 'Group 1'
      | sbobj.Groups.Signals.Name = 'Signal 1'
      | sbobj.Groups.Signals.XData = [0 1.8 2 3.1 3.3 3.9 5 5.8 5.8 6.1 6.1 6.75 10.45 10.45 11.6 11.6 12.6 12.6 13.5 13.5 14.6 14.75 17.95 17.95 18.15 18.6 20]
      | sbobj.Groups.Signals.YData = [-0.01 -0.01 0 0.325 0.615 -0.05 0.2 0.51 0.53 0.53 0.515 -0.14 -0.045 -0.04 0.005 0 -0.045 -0.04 -0.015 -0.02 -0.42 -0.42 0.595 0.61 0.61 0.03 0.03]
      | sbobj.Groups.TimeRange = [0 20]
  Signal 1 : Outport  Tag=STV Outport
  wires:
  FromWs/1 -> Demux/1
  Demux/1 -> Signal 1/1

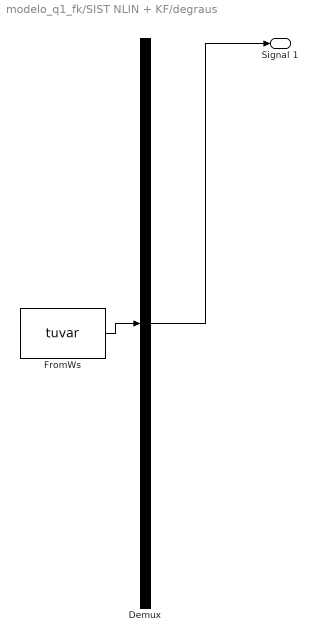
== system modelo_q1_fk/SIST NLIN + KF/degraus ==
  Demux : Demux  Tag=STV Demux  Outputs=1
  FromWs : FromWorkspace  Tag=STV FromWs  VariableName=tuvar  SampleTime=0
      SigBuilderData=|
      | common.afterFinalStr = 'Extrapolate'
      | common.sampleTime = 0
      | dataSet.timeRange = [0 20]
      | dataSet.name = 'Group 1'
      | sbobj.Groups.Name = 'Group 1'
      | sbobj.Groups.Signals.Name = 'Signal 1'
      | sbobj.Groups.Signals.XData = [0 1.8 3.1 3.1 3.3 3.3 3.9 3.9 5.8 5.8 6.1 6.1 6.75 6.75 10.45 10.45 11.6 11.6 12.6 12.6 13.5 13.5 14.6 14.6 14.75 14.75 17.95 17.95 18.15 18.15 18.6 20]
      | sbobj.Groups.Signals.YData = [-0.01 -0.01 -0.01 0.695 0.695 -0.05 -0.05 0 0 0.53 0.53 -0.01 -0.01 -0.14 -0.14 -0.04 -0.04 0 0 -0.04 -0.04 -0.02 -0.02 -0.42 -0.42 -0.01 -0.01 0.61 0.61 0.03 0.03 0.03]
      | sbobj.Groups.TimeRange = [0 20]
  Signal 1 : Outport  Tag=STV Outport
  wires:
  Demux/1 -> Signal 1/1
  FromWs/1 -> Demux/1

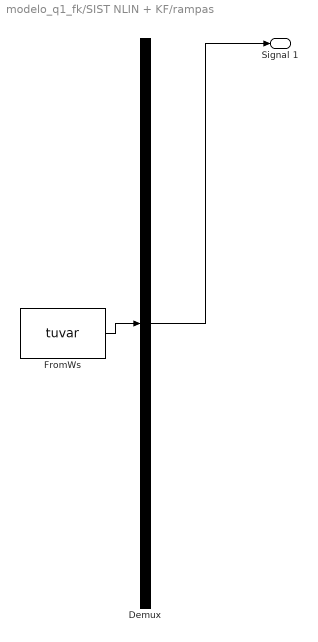
== system modelo_q1_fk/SIST NLIN + KF/rampas ==
  Demux : Demux  Tag=STV Demux  Outputs=1
  FromWs : FromWorkspace  Tag=STV FromWs  VariableName=tuvar  SampleTime=0
      SigBuilderData=|
      | common.afterFinalStr = 'Extrapolate'
      | common.sampleTime = 0
      | dataSet.timeRange = [0 20]
      | dataSet.name = 'Group 1'
      | sbobj.Groups.Name = 'Group 1'
      | sbobj.Groups.Signals.Name = 'Signal 1'
      | sbobj.Groups.Signals.XData = [0 1.8 2 3.1 3.3 3.9 5 5.8 5.8 6.1 6.1 6.75 10.45 10.45 11.6 11.6 12.6 12.6 13.5 13.5 14.6 14.75 17.95 17.95 18.15 18.6 20]
      | sbobj.Groups.Signals.YData = [-0.01 -0.01 0 0.325 0.615 -0.05 0.2 0.51 0.53 0.53 0.515 -0.14 -0.045 -0.04 0.005 0 -0.045 -0.04 -0.015 -0.02 -0.42 -0.42 0.595 0.61 0.61 0.03 0.03]
      | sbobj.Groups.TimeRange = [0 20]
  Signal 1 : Outport  Tag=STV Outport
  wires:
  FromWs/1 -> Demux/1
  Demux/1 -> Signal 1/1

== system modelo_q1_fk/SIST NLIN + KF BLCO/Signal Builder1 ==
  Demux : Demux  Tag=STV Demux  Outputs=1
  FromWs : FromWorkspace  Tag=STV FromWs  VariableName=tuvar  SampleTime=0
      SigBuilderData=|
      | common.afterFinalStr = 'Extrapolate'
      | common.sampleTime = 0
      | dataSet.timeRange = [0 20]
      | dataSet.name = 'Group 1'
      | sbobj.Groups.Name = 'Group 1'
      | sbobj.Groups.Signals.Name = 'Signal 1'
      | sbobj.Groups.Signals.XData = [0 1.8 3.1 3.1 3.3 3.3 3.9 3.9 5.8 5.8 6.1 6.1 6.75 6.75 10.45 10.45 11.6 11.6 12.6 12.6 13.5 13.5 14.6 14.6 14.75 14.75 17.95 17.95 18.15 18.15 18.6 20]
      | sbobj.Groups.Signals.YData = [-0.01 -0.01 -0.01 0.695 0.695 -0.05 -0.05 0 0 0.53 0.53 -0.01 -0.01 -0.14 -0.14 -0.04 -0.04 0 0 -0.04 -0.04 -0.02 -0.02 -0.42 -0.42 -0.01 -0.01 0.61 0.61 0.03 0.03 0.03]
      | sbobj.Groups.TimeRange = [0 20]
  Signal 1 : Outport  Tag=STV Outport
  wires:
  FromWs/1 -> Demux/1
  Demux/1 -> Signal 1/1

== matlab function modelo_q1_fk/SIST NLIN + GANHO FIX/Moto nao linear ==
  data: x1 input; x2 input; x3 input; u input; x1_dot output; x2_dot output; x3_dot output
function [x1_dot, x2_dot, x3_dot] = fcn(x1, x2, x3, u)

mV = 0.152;     % Massa do veículo, sem giroscópio [kg]
mG = 0.15;      % Massa do giroscópio [kg]
rG = 0.095/2;   % Raio do giroscópio [m]
aG = 0.006;     % Espessura do giroscópio [m]
aV = 0.075;     % Altura do veículo [m]
lV = 0.19;      % Comprimento do veículo [m]
dG = 0.06;      % Distância entre centro de massa do giroscópio e centro de rotação do veículo [m]
dV = 0.045;     % Distância entre centro de massa do veículo e o ponto de rotação do veículo [m]

omega = 6500*0.10472;   % Velocidade de rotação do giroscópio, RPM*conversão = rad/sec
g = 9.81;               % Gravidade [m/s^2] 

IG11 = mG*(rG^2)/4 + mG*(aG^2)/12; % Momento de Inércia
IG33 = mG*(rG^2)/2;
IB11 = mV*(aV^2+lV^2)/12; 

num_f3 = (mV*dV+mG*dG)*g*sin(x1);
den_f3 = IB11+mV*dV^2+mG*dG^2+IG11*cos(x2)^2+IG33*sin(x2)^2;
f3 = num_f3/den_f3;

num_u3 = -2*cos(x2)*sin(x2)*(IG33-IG11)*x3-omega*cos(x2)*IG33;
den_u3 = den_f3;
u3 = num_u3/den_u3;

x1_dot = x3;
x2_dot = u;
x3_dot = f3+u3*u;

== matlab function modelo_q1_fk/SIST NLIN + KF BLCO/Moto nao linear ==
  data: x1 input; x2 input; x3 input; u input; x1_dot output; x2_dot output; x3_dot output
function [x1_dot, x2_dot, x3_dot] = fcn(x1, x2, x3, u)

mV = 0.152;     % Massa do veículo, sem giroscópio [kg]
mG = 0.15;      % Massa do giroscópio [kg]
rG = 0.095/2;   % Raio do giroscópio [m]
aG = 0.006;     % Espessura do giroscópio [m]
aV = 0.075;     % Altura do veículo [m]
lV = 0.19;      % Comprimento do veículo [m]
dG = 0.06;      % Distância entre centro de massa do giroscópio e centro de rotação do veículo [m]
dV = 0.045;     % Distância entre centro de massa do veículo e o ponto de rotação do veículo [m]

omega = 6500*0.10472;   % Velocidade de rotação do giroscópio, RPM*conversão = rad/sec
g = 9.81;               % Gravidade [m/s^2] 

IG11 = mG*(rG^2)/4 + mG*(aG^2)/12; % Momento de Inércia
IG33 = mG*(rG^2)/2;
IB11 = mV*(aV^2+lV^2)/12; 

num_f3 = (mV*dV+mG*dG)*g*sin(x1);
den_f3 = IB11+mV*dV^2+mG*dG^2+IG11*cos(x2)^2+IG33*sin(x2)^2;
f3 = num_f3/den_f3;

num_u3 = -2*cos(x2)*sin(x2)*(IG33-IG11)*x3-omega*cos(x2)*IG33;
den_u3 = den_f3;
u3 = num_u3/den_u3;

x1_dot = x3;
x2_dot = u;
x3_dot = f3+u3*u;

== matlab function modelo_q1_fk/SIST NLIN + EKF/Extended KF ==
  data: x1a input; x2a input; x3a input; Pa input; u input; x1 output; y input; Ts input; x2 output; x3 output; Pa output; C input; w input; v input
function [x1,x2,x3,Pa] = kalman(x1a,x2a,x3a,Pa,u,y,Ts,C,w,v)



% Parâmetros do modelo
Mv = 0.152; % Massa do veículo sem giro [kg]
Mg = 0.15; % Massa do giro [kg]
Rg = 0.095/2; % Raio do giro [m]
Ag = 0.006; % Es  pessura giro [m]
Av = 0.075; % Altura veículo [m]
Lv = 0.19; % Largura veículo [m]
Dg = 0.06; % Distância entre centro de massa do giro e eixo de rotação [m]
Dv = 0.045; % Distância entre centro de massa do veículo e eixo de rotação
Omega = 6500*0.10472; % Velocidade de rotação do giro, rpm*conversão = rad/sec
g = 9.81; % Gravidade [m/s^2] 
IG11 = (Mg*(Rg^2)/4) + (Mg*(Ag^2)/12); % Algum momento de inercia
IG33 = Mg*(Rg^2)/2;
IB11 = Mv*(Av^2+Lv^2)/12; 

%funcao nao linear
f1 = x3a;
f2 = 0;
f3 = ((Mv*Dv+Mg*Dg)*g*sin(x1a))/(IB11+Mv*(Dv^2)+IG11*(cos(x2a)^2)+Mg*(Dg^2)+IG33*((sin(x2a))^2));
f = [f1;f2;f3];
g1 = 0;
g2 = 1;
g3 = (-2*cos(x2a)*sin(x2a)*x3a*(IG33-IG11)-Omega*cos(x2a)*IG33)/(IB11+IG11*(cos(x2a)^2)+Mv*(Dv^2)+Mg*(Dg^2)+IG33*(sin(x2a)^2));
g=[g1;g2;g3];

%x1a, x2a, x3a = x k-1|k-1
%jacobiano de f e g
f31 = -(35830586753891961600000*cos(x1a))/(19405830650354371875*cos(x2a)^2 - 356376203601300673408);
f32 = -(1390644597297715974832459795959240000000000*cos(x2a)*sin(x1a)*sin(x2a))/(19405830650354371875*sin(x2a)^2 + 336970372950946301533)^2;
f_jac = [ 0 0 1;
          0 0 0;
      f31 f32 0];
g32 = -(13078379983345635015350619020697129168750*x3a - 9980613122993816581722710681833220711909000*sin(x2a) - 26909932493151736398074981075245840368750*x3a*sin(x2a)^2 + 515410717910523541987644337581435553125000*sin(x2a)^3)/(19405830650354371875*sin(x2a)^2 + 336970372950946301533)^2;
g33 = (19405830650354371875*sin(2*x2a))/((19405830650354371875*cos(2*x2a))/2 - 693346576552246974941/2);
g_jac = [0 0 0;
         0 0 0; 
         0 g32 g33];

%xa = x k|k-1
xa = f+g*u;%+diag(w);

%A =(f_jac+g_jac*u);
A =(f_jac+g_jac*u)*Ts*1e3 + eye(3);

%PREVISAO
%xp = A*x+B*u;
xc = [x1a;x2a;x3a];
%xp = A*xc+g*u;
Pp = (A*Pa)*transpose(A) + w;
K = Pp*transpose(C)/(C*Pp*transpose(C)+v);
x = xa+ K*(y-C*xa);
% x => x k|k
Pa = (eye(3)-K*C)*Pp;
x1 = x(1,1);
x2 = x(2,1);
x3 = x(3,1);

end

== matlab function modelo_q1_fk/SIST NLIN + KF/Moto nao linear ==
  data: x1 input; x2 input; x3 input; u input; x1_dot output; x2_dot output; x3_dot output
function [x1_dot, x2_dot, x3_dot] = fcn(x1, x2, x3, u)

mV = 0.152;     % Massa do veículo, sem giroscópio [kg]
mG = 0.15;      % Massa do giroscópio [kg]
rG = 0.095/2;   % Raio do giroscópio [m]
aG = 0.006;     % Espessura do giroscópio [m]
aV = 0.075;     % Altura do veículo [m]
lV = 0.19;      % Comprimento do veículo [m]
dG = 0.06;      % Distância entre centro de massa do giroscópio e centro de rotação do veículo [m]
dV = 0.045;     % Distância entre centro de massa do veículo e o ponto de rotação do veículo [m]

omega = 6500*0.10472;   % Velocidade de rotação do giroscópio, RPM*conversão = rad/sec
g = 9.81;               % Gravidade [m/s^2] 

IG11 = mG*(rG^2)/4 + mG*(aG^2)/12; % Momento de Inércia
IG33 = mG*(rG^2)/2;
IB11 = mV*(aV^2+lV^2)/12; 

num_f3 = (mV*dV+mG*dG)*g*sin(x1);
den_f3 = IB11+mV*dV^2+mG*dG^2+IG11*cos(x2)^2+IG33*sin(x2)^2;
f3 = num_f3/den_f3;

num_u3 = -2*cos(x2)*sin(x2)*(IG33-IG11)*x3-omega*cos(x2)*IG33;
den_u3 = den_f3;
u3 = num_u3/den_u3;

x1_dot = x3;
x2_dot = u;
x3_dot = f3+u3*u;

== matlab function modelo_q1_fk/SIST NLIN + KF/KF ==
  data: x1a input; x2a input; x3a input; Pa input; u input; x1 output; y input; x2 output; x3 output; Pa output; A input; B input; C input; w input; v input
    function [x1,x2,x3,Pa] = kalman(x1a,x2a,x3a,Pa,u,y,A,B,C,w,v)

x1 = x1a;
x2 = x2a;
x3 = x3a;

%PREVISAO
%xp = A*x+B*u;
x1p = A(1,1)*x1+A(1,2)*x2+A(1,3)*x3+B(1,1)*u +w(1,1);
x2p = A(2,1)*x1+A(2,2)*x2+A(2,3)*x3+B(2,1)*u+w(2,2);
x3p = A(3,1)*x1+A(3,2)*x2+A(3,3)*x3+B(3,1)*u+w(3,3);

Pp = (A*Pa)*transpose(A) + w;
xp = [x1p;x2p;x3p];
K = Pp*transpose(C)/(C*Pp*transpose(C)+v);
x = xp + K*(y-C*xp);
Pa = (eye(3)-K*C)*Pp;
x1 = x(1,1);
x2 = x(2,1);
x3 = x(3,1);

end

== matlab function modelo_q1_fk/SIST NLIN + EKF/Moto nao linear ==
  data: x1 input; x2 input; x3 input; u input; x1_dot output; x2_dot output; x3_dot output
function [x1_dot, x2_dot, x3_dot] = fcn(x1, x2, x3, u)

mV = 0.152;     % Massa do veículo, sem giroscópio [kg]
mG = 0.15;      % Massa do giroscópio [kg]
rG = 0.095/2;   % Raio do giroscópio [m]
aG = 0.006;     % Espessura do giroscópio [m]
aV = 0.075;     % Altura do veículo [m]
lV = 0.19;      % Comprimento do veículo [m]
dG = 0.06;      % Distância entre centro de massa do giroscópio e centro de rotação do veículo [m]
dV = 0.045;     % Distância entre centro de massa do veículo e o ponto de rotação do veículo [m]

omega = 6500*0.10472;   % Velocidade de rotação do giroscópio, RPM*conversão = rad/sec
g = 9.81;               % Gravidade [m/s^2] 

IG11 = mG*(rG^2)/4 + mG*(aG^2)/12; % Momento de Inércia
IG33 = mG*(rG^2)/2;
IB11 = mV*(aV^2+lV^2)/12; 

num_f3 = (mV*dV+mG*dG)*g*sin(x1);
den_f3 = IB11+mV*dV^2+mG*dG^2+IG11*cos(x2)^2+IG33*sin(x2)^2;
f3 = num_f3/den_f3;

num_u3 = -2*cos(x2)*sin(x2)*(IG33-IG11)*x3-omega*cos(x2)*IG33;
den_u3 = den_f3;
u3 = num_u3/den_u3;

x1_dot = x3;
x2_dot = u;
x3_dot = f3+u3*u;

== matlab function modelo_q1_fk/SIST NLIN + GANHO FIX1/Moto nao linear ==
  data: x1 input; x2 input; x3 input; u input; x1_dot output; x2_dot output; x3_dot output
function [x1_dot, x2_dot, x3_dot] = fcn(x1, x2, x3, u)

mV = 0.152;     % Massa do veículo, sem giroscópio [kg]
mG = 0.15;      % Massa do giroscópio [kg]
rG = 0.095/2;   % Raio do giroscópio [m]
aG = 0.006;     % Espessura do giroscópio [m]
aV = 0.075;     % Altura do veículo [m]
lV = 0.19;      % Comprimento do veículo [m]
dG = 0.06;      % Distância entre centro de massa do giroscópio e centro de rotação do veículo [m]
dV = 0.045;     % Distância entre centro de massa do veículo e o ponto de rotação do veículo [m]

omega = 6500*0.10472;   % Velocidade de rotação do giroscópio, RPM*conversão = rad/sec
g = 9.81;               % Gravidade [m/s^2] 

IG11 = mG*(rG^2)/4 + mG*(aG^2)/12; % Momento de Inércia
IG33 = mG*(rG^2)/2;
IB11 = mV*(aV^2+lV^2)/12; 

num_f3 = (mV*dV+mG*dG)*g*sin(x1);
den_f3 = IB11+mV*dV^2+mG*dG^2+IG11*cos(x2)^2+IG33*sin(x2)^2;
f3 = num_f3/den_f3;

num_u3 = -2*cos(x2)*sin(x2)*(IG33-IG11)*x3-omega*cos(x2)*IG33;
den_u3 = den_f3;
u3 = num_u3/den_u3;

x1_dot = x3;
x2_dot = u;
x3_dot = f3+u3*u;

== matlab function modelo_q1_fk/SIST NLIN + GANHO FIX1/Extended KF ==
  data: x1a input; x2a input; x3a input; Pa input; u input; x1 output; y input; Ts input; x2 output; x3 output; Pa output; C input; w input; v input
function [x1,x2,x3,Pa] = kalman(x1a,x2a,x3a,Pa,u,y,Ts,C,w,v)



% Parâmetros do modelo
Mv = 0.152; % Massa do veículo sem giro [kg]
Mg = 0.15; % Massa do giro [kg]
Rg = 0.095/2; % Raio do giro [m]
Ag = 0.006; % Es  pessura giro [m]
Av = 0.075; % Altura veículo [m]
Lv = 0.19; % Largura veículo [m]
Dg = 0.06; % Distância entre centro de massa do giro e eixo de rotação [m]
Dv = 0.045; % Distância entre centro de massa do veículo e eixo de rotação
Omega = 6500*0.10472; % Velocidade de rotação do giro, rpm*conversão = rad/sec
g = 9.81; % Gravidade [m/s^2] 
IG11 = (Mg*(Rg^2)/4) + (Mg*(Ag^2)/12); % Algum momento de inercia
IG33 = Mg*(Rg^2)/2;
IB11 = Mv*(Av^2+Lv^2)/12; 

%funcao nao linear
f1 = x3a;
f2 = 0;
f3 = ((Mv*Dv+Mg*Dg)*g*sin(x1a))/(IB11+Mv*(Dv^2)+IG11*(cos(x2a)^2)+Mg*(Dg^2)+IG33*((sin(x2a))^2));
f = [f1;f2;f3];
g1 = 0;
g2 = 1;
g3 = (-2*cos(x2a)*sin(x2a)*x3a*(IG33-IG11)-Omega*cos(x2a)*IG33)/(IB11+IG11*(cos(x2a)^2)+Mv*(Dv^2)+Mg*(Dg^2)+IG33*(sin(x2a)^2));
g=[g1;g2;g3];

%x1a, x2a, x3a = x k-1|k-1
%jacobiano de f e g
f31 = -(35830586753891961600000*cos(x1a))/(19405830650354371875*cos(x2a)^2 - 356376203601300673408);
f32 = -(1390644597297715974832459795959240000000000*cos(x2a)*sin(x1a)*sin(x2a))/(19405830650354371875*sin(x2a)^2 + 336970372950946301533)^2;
f_jac = [ 0 0 1;
          0 0 0;
      f31 f32 0];
g32 = -(13078379983345635015350619020697129168750*x3a - 9980613122993816581722710681833220711909000*sin(x2a) - 26909932493151736398074981075245840368750*x3a*sin(x2a)^2 + 515410717910523541987644337581435553125000*sin(x2a)^3)/(19405830650354371875*sin(x2a)^2 + 336970372950946301533)^2;
g33 = (19405830650354371875*sin(2*x2a))/((19405830650354371875*cos(2*x2a))/2 - 693346576552246974941/2);
g_jac = [0 0 0;
         0 0 0; 
         0 g32 g33];

%xa = x k|k-1
xa = f+g*u%+diag(w);

%A =(f_jac+g_jac*u);
A =(f_jac+g_jac*u)*Ts;% + eye(3)

%PREVISAO
%xp = A*x+B*u;
xc = [x1a;x2a;x3a];

%xp = A*xc+g*u;

Pp = (A*Pa)*transpose(A) + w;
K = Pp*transpose(C)/(C*Pp*transpose(C)+v);

% x => x k|k
x = xa+ K*(y-C*xa);

Pa = (eye(3)-K*C)*Pp;

x1 = x(1,1);
x2 = x(2,1);
x3 = x(3,1);

end
